simulink model "c"  (R2018b)
settings: Solver=FixedStepAuto  StartTime=0.0  StopTime=10.68  FixedStep=0.01  RelTol=1e-3
settings Model: Creator=yizha  LastModifiedBy=yizha

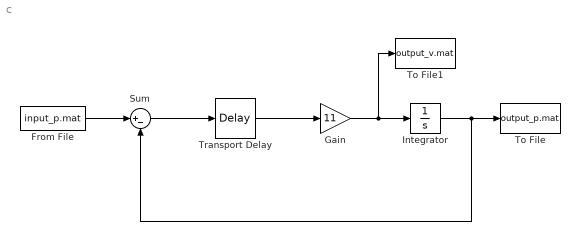
== system c ==
  From File : FromFile  FileName=input_p.mat  SampleTime=0
  Gain : Gain  Gain=11
  Integrator : Integrator
  Sum : Sum  Inputs=|+-
  To File : ToFile  Filename=output_p.mat
  To File1 : ToFile  Filename=output_v.mat
  Transport Delay : TransportDelay  DelayTime=0.1
  wires:
  Integrator/1 -> To File/1, Sum/2
  Sum/1 -> Transport Delay/1
  Transport Delay/1 -> Gain/1
  Gain/1 -> To File1/1, Integrator/1
  From File/1 -> Sum/1
